simulink model "F28379DFirmware"  (R2026a)
settings: Solver=FixedStepAuto  StopTime=Inf  FixedStep=5e-5  EnableMultiTasking=on
undefined symbols (not defined in the file): bit, DiscIntNeverNeededParam, Down, F28379D_ADC_MaxCount, F28379D_ADC_Vmax, F28379D_PWM_Counter_Period, Foc_Ki_IxTcpu, Foc_Ki_S, Foc_Kp_I, Foc_Kp_S, GPTRIP1SEL, GPTRIP2SEL, Ia_offset, Ib_offset, IO334_DAC_Vmax, Maxon_645604_Np, PU_System_I_base, PU_System_N_base, Ts_CPU, TZ1, TZ2, Up
libraries: c280xlib x8, mcbcontrolslib x8, canmsglib x7, c2802xlib x6, mcbeeMathTransformLib x3, slpidlib x3, simulink x3, mcbpositiondecoderlib x3, c2837xDlib x3, demo_controls x1
(part 2 of 2)

== system F28379DFirmware/F28379D Firmware/Controller Algorithm/FOC/Speed Control MLD ==
  En_closedloop : Inport
  EnablePWM : Inport  Port=2
  SpeedRef : Inport  Port=3
  Speed_Meas_PU : Inport  Port=4
  Kp_S : Inport  Port=5
  Ki_S : Inport  Port=6
  AND : Logic  IconShape=distinctive  AllPortsSameDT=off  OutDataTypeStr=boolean
  Id_Ref : Constant  Value=0  OutDataTypeStr=single
  Mux : Mux  Inputs=2
  PI_Controller_Speed : Subsystem
  Speed_Ref_Selector : Subsystem
  IdqRef_PU : Outport  VectorParamsAs1DForOutWhenUnconnected=off
  wires:
  Mux/1 -> IdqRef_PU/1
  En_closedloop/1 -> AND/1, PI_Controller_Speed/1(Enable)
  Kp_S/1 -> PI_Controller_Speed/4(Kp_S)
  EnablePWM/1 -> AND/2
  Speed_Ref_Selector/1(Speed_Ref_PU) -> PI_Controller_Speed/2(N_ref)
  PI_Controller_Speed/1(Iq_ref) -> Mux/2
  SpeedRef/1 -> Speed_Ref_Selector/2(SpeedCommand)
  AND/1 -> Speed_Ref_Selector/1(Enable)
  Speed_Meas_PU/1 -> PI_Controller_Speed/3(N_fb), Speed_Ref_Selector/3(Speed_Ref_Open)
  Id_Ref/1 -> Mux/1
  Ki_S/1 -> PI_Controller_Speed/5(Ki_S)

== system F28379DFirmware/F28379D Firmware/Controller Algorithm/Speed and Pos Decoder/IndexFinder ==
  In1 : Inport
  Enable : EnablePort
  AND : Logic  AllPortsSameDT=off  OutDataTypeStr=boolean
  Compare To Constant : simulink/Logic and Bit Operations/Compare To Constant  relop===  const=0  OutDataTypeStr=boolean
  Compare To Constant1 : simulink/Logic and Bit Operations/Compare To Constant  relop=>  const=0  OutDataTypeStr=boolean
  Delay3 : Delay  DelayLength=1
  IndexFound : Outport
  wires:
  In1/1 -> Delay3/1, Compare To Constant1/1
  Compare To Constant1/1 -> AND/2
  Compare To Constant/1 -> AND/1
  Delay3/1 -> Compare To Constant/1
  AND/1 -> IndexFound/1

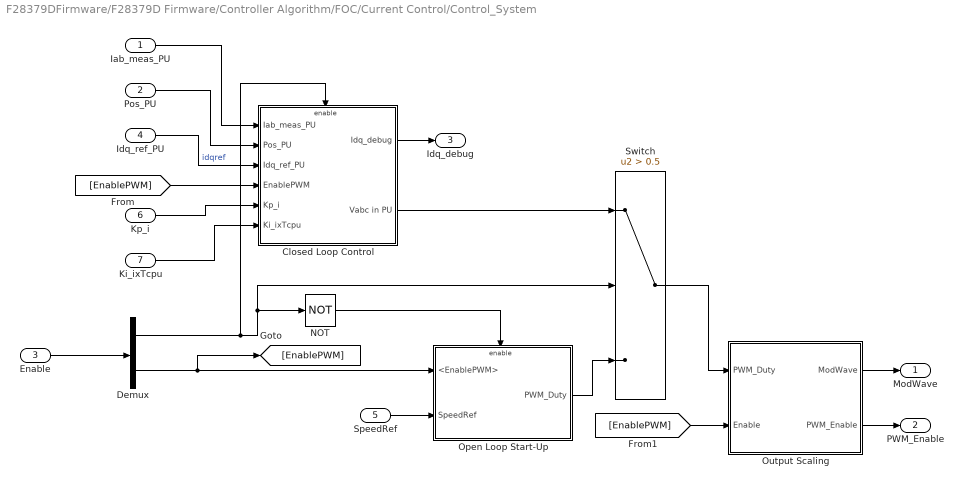
== system F28379DFirmware/F28379D Firmware/Controller Algorithm/FOC/Current Control/Control_System ==
  Iab_meas_PU : Inport
  Pos_PU : Inport  Port=2
  Enable : Inport  Port=3
  Idq_ref_PU : Inport  Port=4
  SpeedRef : Inport  Port=5
  Kp_i : Inport  Port=6
  Ki_ixTcpu : Inport  Port=7
  Closed Loop Control : Subsystem
  Demux : Demux  Outputs=2
  NOT : Logic  Operator=NOT  IconShape=distinctive  AllPortsSameDT=off  OutDataTypeStr=boolean
  Open Loop Start-Up : Subsystem
  Output Scaling : Subsystem
  Switch : Switch  Criteria=u2 > Threshold  Threshold=0.5  SaturateOnIntegerOverflow=off  InputSameDT=off
  ModWave : Outport
  PWM_Enable : Outport  Port=2
  Idq_debug : Outport  Port=3  VectorParamsAs1DForOutWhenUnconnected=off
  wires:
  Enable/1 -> Demux/1
  Idq_ref_PU/1 -> Closed Loop Control/3(Idq_ref_PU)  "idqref"
  Demux/2 -> [EnablePWM], Open Loop Start-Up/1(<EnablePWM>)
  [EnablePWM] -> Closed Loop Control/4(EnablePWM)
  Demux/1 -> Switch/2, NOT/1, Closed Loop Control/Enable
  Iab_meas_PU/1 -> Closed Loop Control/1(Iab_meas_PU)
  Pos_PU/1 -> Closed Loop Control/2(Pos_PU)
  SpeedRef/1 -> Open Loop Start-Up/2(SpeedRef)
  Kp_i/1 -> Closed Loop Control/5(Kp_i)
  Ki_ixTcpu/1 -> Closed Loop Control/6(Ki_ixTcpu)
  Closed Loop Control/2(Vabc in PU) -> Switch/1
  Closed Loop Control/1(Idq_debug) -> Idq_debug/1
  NOT/1 -> Open Loop Start-Up/Enable
  Open Loop Start-Up/1(PWM_Duty) -> Switch/3
  Switch/1 -> Output Scaling/1(PWM_Duty)
  [EnablePWM] -> Output Scaling/2(Enable)
  Output Scaling/2(PWM_Enable) -> PWM_Enable/1
  Output Scaling/1(ModWave) -> ModWave/1

== system F28379DFirmware/F28379D Firmware/Controller Algorithm/FOC/Speed Control MLD/PI_Controller_Speed ==
  Enable : Inport
  N_ref : Inport  Port=2
  N_fb : Inport  Port=3
  Kp_S : Inport  Port=4
  Ki_S : Inport  Port=5
  Discrete PI Controller with anti-windup & reset : slpidlib/PID Controller  Controller=PI  Form=Parallel  TimeDomain=Discrete-time  UseExternalTs=off  SampleTime=-1  IntegratorMethod=Forward Euler  FilterMethod=Forward Euler  ControllerParametersSource=external  P=1  I=1  UseKiTs=on  D=0  UseExternalDerivativeSource=off  N=100  UseFilter=on  TunerSelectOption=Transfer Function Based (PID Tuner App)  InitialConditionSource=external  InitialConditionForIntegrator=0  InitialConditionForFilter=0  DifferentiatorICPrevScaledInput=0  ExternalReset=level  TrackingMode=off  Kt=1  LimitOutput=on  SatLimitsSource=internal  UpperSaturationLimit=1  LowerSaturationLimit=-1  LinearizeAsGain=on  AntiWindupMode=clamping  Kb=1  LimitIntegrator=off  UpperIntegratorSaturationLimit=inf  LowerIntegratorSaturationLimit=-inf  RndMeth=Simplest  POutMin=[]  POutMax=[]  IOutMin=[]  IOutMax=[]  DOutMin=[]  DOutMax=[]  NOutMin=[]  NOutMax=[]  SumOutMin=[]  SumOutMax=[]  SaturationOutDataTypeStr=Inherit: Inherit via back propagation  SaturationOutMin=[]  SaturationOutMax=[]  PParamMin=[]  PParamMax=[]  IParamMin=[]  IParamMax=[]  DParamMin=[]  DParamMax=[]  NParamMin=[]  NParamMax=[]  KbParamMin=[]  KbParamMax=[]  KtParamMin=[]  KtParamMax=[]  KbOutMin=[]  KbOutMax=[]  KtOutMin=[]  KtOutMax=[]  IntegratorOutMin=[]  IntegratorOutMax=[]  FilterOutMin=[]  FilterOutMax=[]  SumI1OutMin=[]  SumI1OutMax=[]  SumI2OutMin=[]  SumI2OutMax=[]  SumI3OutMin=[]  SumI3OutMax=[]  SumI4OutMin=[]  SumI4OutMax=[]  SumDOutMin=[]  SumDOutMax=[]  DifferentiatorOutMin=[]  DifferentiatorOutMax=[]  FilterDiffOutCoefMin=[]  FilterDiffOutCoefMax=[]  ReciprocalOutMin=[]  ReciprocalOutMax=[]  SumDenOutMin=[]  SumDenOutMax=[]  SumNumOutMin=[]  SumNumOutMax=[]  DivideOutMin=[]  DivideOutMax=[]  UdiffTsProdOutMin=[]  UdiffTsProdOutMax=[]  NTsProdOutMin=[]  NTsProdOutMax=[]  UintegralTsProdOutMin=[]  UintegralTsProdOutMax=[]  UngainTsProdOutMin=[]  UngainTsProdOutMax=[]  ClampingZeroOutDataTypeStr=Inherit: Inherit via back propagation  ClampingZeroOutMin=[]  ClampingZeroOutMax=[]  FilterDenConstantOutDataTypeStr=Inherit: Inherit via back propagation  FilterDenConstantOutMin=[]  FilterDenConstantOutMax=[]  PCopyOutDataTypeStr=Inherit: Inherit via back propagation  PCopyOutMin=[]  PCopyOutMax=[]  NCopyOutDataTypeStr=Inherit: Inherit via back propagation  NCopyOutMin=[]  NCopyOutMax=[]  IntegratorContinuousStateAttributes=''  IntegratorStateMustResolveToSignalObject=off  IntegratorRTWStateStorageClass=Auto  FilterContinuousStateAttributes=''  FilterStateMustResolveToSignalObject=off  FilterRTWStateStorageClass=Auto  ParallelPVariant=ExternalParameters  IdealPVariant=Disabled  IVariant=ExternalParameters  DVariant=Disabled  IntegratorVariant=Discrete  SatVariant=Enabled  AWVariant=DiscClampingParallel  PCopyVariant=Disabled  TRVariant=Disabled  FdbkBlocksVariant=Forward  IdealPFdbkVariant=Disabled  SatFdbkVariant=Disabled  DerivativeFilterVariant=Disabled  NVariant=Disabled  NCopyVariant=Disabled_SignalSpec  FilterICVariant=Disabled  IntegratorICVariant=ExternalICs  ExternalResetVariant=ExternalReset  TRSumVariant=Passthrough  SumFdbkVariant=Disabled  SumVariant=Sum_PI  TsampFilterVariant=InternalTs  TsampNgainVariant=Passthrough  TsampIntegralVariant=Disabled_SignalSpec  ExternalSaturationOutDataTypeStr=Inherit: Same as second input  DerivativeSourceVariant=Disabled  PreIntVariant=InternalPreInt
  Ki2 : Constant  Value=0  OutDataTypeStr=single  SampleTime=-1
  Logical Operator : Logic  Operator=NOT  IconShape=distinctive  AllPortsSameDT=off  OutDataTypeStr=boolean
  Sum : Sum  Inputs=|+-  OutDataTypeStr=Inherit: Same as first input
  Iq_ref : Outport  VectorParamsAs1DForOutWhenUnconnected=off
  wires:
  Ki_S/1 -> Discrete PI Controller with anti-windup & reset/3
  Kp_S/1 -> Discrete PI Controller with anti-windup & reset/2
  Enable/1 -> Logical Operator/1
  Ki2/1 -> Discrete PI Controller with anti-windup & reset/5
  Logical Operator/1 -> Discrete PI Controller with anti-windup & reset/4
  Sum/1 -> Discrete PI Controller with anti-windup & reset/1
  N_ref/1 -> Sum/1
  N_fb/1 -> Sum/2
  Discrete PI Controller with anti-windup & reset/1 -> Iq_ref/1

== system F28379DFirmware/F28379D Firmware/Controller Algorithm/FOC/Speed Control MLD/Speed_Ref_Selector ==
  Enable : Inport
  SpeedCommand : Inport  Port=2
  Speed_Ref_Open : Inport  Port=3
  IIR Filter : mcbcontrolslib/IIR Filter  VariantControl=Low Pass Filter  VariantSelect=Low-pass  FilterConstantInputType=Specify via dialog  Filter_constant=0.01  InitialOutput=Specify via dialog  InitialOutputValue=0  ExternalReset=none  advancedSettings=off  Ts=50e-6  cutOff_freq=32.1525
  Switch : Switch  Criteria=u2 > Threshold  Threshold=0.5  SaturateOnIntegerOverflow=off  InputSameDT=off
  Speed_Ref_PU : Outport
  wires:
  SpeedCommand/1 -> Switch/1  "SpeedRef"
  Enable/1 -> Switch/2
  Speed_Ref_Open/1 -> Switch/3
  Switch/1 -> IIR Filter/1
  IIR Filter/1 -> Speed_Ref_PU/1

== system F28379DFirmware/F28379D Firmware/Controller Algorithm/FOC/Current Control/Control_System/Closed Loop Control ==
  Iab_meas_PU : Inport
  Pos_PU : Inport  Port=2
  Idq_ref_PU : Inport  Port=3
  EnablePWM : Inport  Port=4
  Kp_i : Inport  Port=5
  Ki_ixTcpu : Inport  Port=6
  Enable : EnablePort
  Subsystem : Subsystem
  Terminator : Terminator
  Idq_debug : Outport
  Vabc in PU : Outport  Port=2
  wires:
  Subsystem/3(VI_fb) -> Terminator/1
  Idq_ref_PU/1 -> Subsystem/3(Idq_ref_PU)
  Iab_meas_PU/1 -> Subsystem/1(Iab_meas_PU)
  EnablePWM/1 -> Subsystem/4(EnablePWM)
  Pos_PU/1 -> Subsystem/2(Pos_PU)
  Subsystem/2(VIdq_debug) -> Idq_debug/1
  Subsystem/1(Vabc in PU) -> Vabc in PU/1
  Ki_ixTcpu/1 -> Subsystem/6(Ki_ixTcpu)
  Kp_i/1 -> Subsystem/5(Kp_i)

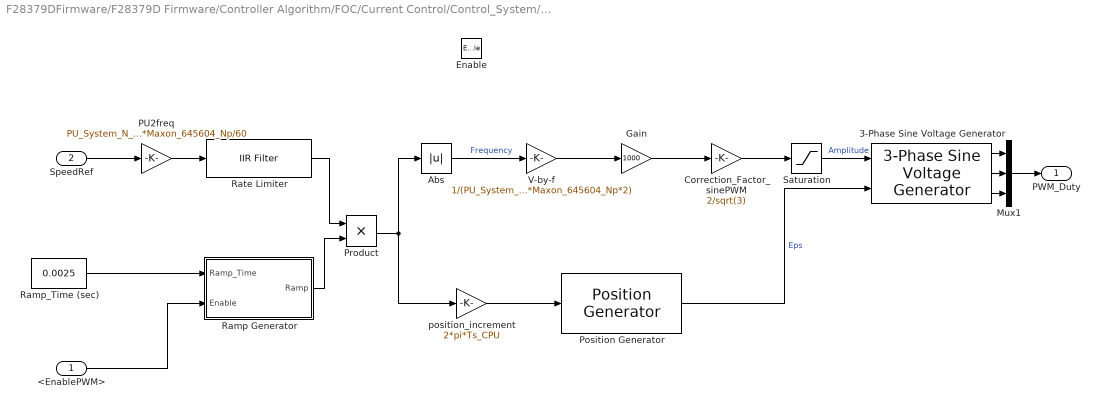
== system F28379DFirmware/F28379D Firmware/Controller Algorithm/FOC/Current Control/Control_System/Open Loop Start-Up ==
  <EnablePWM> : Inport
  SpeedRef : Inport  Port=2
  Enable : EnablePort
  3-Phase Sine Voltage Generator : mcbcontrolslib/3-Phase Sine Voltage Generator  AngleInput=Radians  N_points=1024
  Abs : Abs  SaturateOnIntegerOverflow=off
  Correction_Factor_sinePWM : Gain  Gain=2/sqrt(3)  RndMeth=Simplest  OutDataTypeStr=Inherit: Same as input
  Gain : Gain  Gain=1000
  Mux1 : Mux  Inputs=3
  PU2freq : Gain  Gain=PU_System_N_base *Maxon_645604_Np/60  RndMeth=Simplest  OutDataTypeStr=Inherit: Same as input
  Position Generator : mcbcontrolslib/Position Generator  AngleOutput=Radians  InitialThetaSource=Specify via dialog  ExternalReset=none  Offset=0
  Product : Product  RndMeth=Simplest  OutDataTypeStr=Inherit: Same as first input
  Ramp Generator : Subsystem
  Ramp_Time (sec) : Constant  Value=0.0025  OutDataTypeStr=single  SampleTime=-1
  Rate Limiter : mcbcontrolslib/IIR Filter  VariantControl=Low Pass Filter  VariantSelect=Low-pass  FilterConstantInputType=Specify via dialog  Filter_constant=0.0001  InitialOutput=Specify via dialog  InitialOutputValue=0  ExternalReset=none  advancedSettings=off  Ts=50e-6  cutOff_freq=0.31834
  Saturation : Saturate  UpperLimit=0.95  LowerLimit=0.15  RndMeth=Simplest
  V-by-f : Gain  Gain=1/(PU_System_N_base*Maxon_645604_Np*2)  RndMeth=Simplest  OutDataTypeStr=Inherit: Same as input
  position_increment : Gain  Gain=2*pi*Ts_CPU  RndMeth=Simplest  OutDataTypeStr=Inherit: Same as input
  PWM_Duty : Outport  VectorParamsAs1DForOutWhenUnconnected=off
  wires:
  3-Phase Sine Voltage Generator/1 -> Mux1/1
  3-Phase Sine Voltage Generator/3 -> Mux1/3
  Position Generator/1 -> 3-Phase Sine Voltage Generator/2  "Eps"
  Saturation/1 -> 3-Phase Sine Voltage Generator/1  "Amplitude"
  Mux1/1 -> PWM_Duty/1
  Ramp Generator/1(Ramp) -> Product/2
  Ramp_Time (sec)/1 -> Ramp Generator/1(Ramp_Time)
  Abs/1 -> V-by-f/1  "Frequency"
  position_increment/1 -> Position Generator/1
  V-by-f/1 -> Gain/1
  PU2freq/1 -> Rate Limiter/1
  Correction_Factor_sinePWM/1 -> Saturation/1
  3-Phase Sine Voltage Generator/2 -> Mux1/2
  <EnablePWM>/1 -> Ramp Generator/2(Enable)
  Product/1 -> Abs/1, position_increment/1
  Rate Limiter/1 -> Product/1
  SpeedRef/1 -> PU2freq/1
  Gain/1 -> Correction_Factor_sinePWM/1

== system F28379DFirmware/F28379D Firmware/Controller Algorithm/FOC/Current Control/Control_System/Output Scaling ==
  PWM_Duty : Inport
  Enable : Inport  Port=2
  Constant : Constant  Value=0.5  OutDataTypeStr=single
  Data Type Conversion : DataTypeConversion  OutDataTypeStr=single  SaturateOnIntegerOverflow=off  RndMeth=Floor
  Gain : Gain  Gain=0.5  OutDataTypeStr=Inherit: Same as input
  Sum : Sum  Inputs=|++
  ModWave : Outport
  PWM_Enable : Outport  Port=2
  wires:
  Sum/1 -> ModWave/1  "duty"
  Constant/1 -> Sum/2
  Gain/1 -> Sum/1  "ModWave"
  PWM_Duty/1 -> Gain/1
  Data Type Conversion/1 -> PWM_Enable/1
  Enable/1 -> Data Type Conversion/1

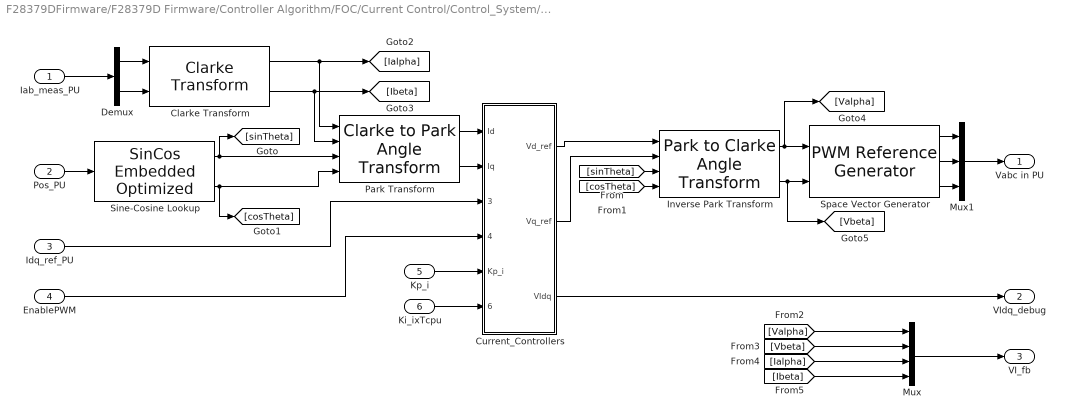
== system F28379DFirmware/F28379D Firmware/Controller Algorithm/FOC/Current Control/Control_System/Closed Loop Control/Subsystem ==
  Iab_meas_PU : Inport
  Pos_PU : Inport  Port=2
  Idq_ref_PU : Inport  Port=3
  EnablePWM : Inport  Port=4
  Kp_i : Inport  Port=5
  Ki_ixTcpu : Inport  Port=6
  Clarke Transform : mcbeeMathTransformLib/Clarke Transform  VariantControl=Variant2  PowerInvariant=off  UseWithEmbedded=on  PhaseInput=Two inputs
      settings: LibrarySourceBlock=mcbcontrolslib/Clarke Transform
  Current_Controllers : Subsystem
  Demux : Demux  Outputs=2
  Inverse Park Transform : mcbeeMathTransformLib/Park to Clarke Angle Transform  AxisAlignment=D-axis  UseWithEmbedded=on  PhaseInput=Two inputs  ThetaInput=Sine and Cosine electrical position  AngleInput=Per-unit  N_points=1024
      settings: LibrarySourceBlock=mcbcontrolslib/Inverse Park Transform
  Mux : Mux
  Mux1 : Mux  Inputs=3
  Park Transform : mcbeeMathTransformLib/Clarke to Park Angle Transform  AxisAlignment=D-axis  UseWithEmbedded=on  PhaseInput=Two inputs  ThetaInput=Sine and Cosine electrical position  AngleInput=Per-unit  N_points=1024
      settings: LibrarySourceBlock=mcbcontrolslib/Park Transform
  Sine-Cosine Lookup : mcbcontrolslib/SinCos Embedded Optimized  LabelModeActiveChoice=MCB_Sin  OptforProc=off  OptLevelPop=Disabled  ApproximationMethod=None  UserApproxMethod=Lookup  ApproxStatus=None  ThetaDataType=double  CopyThetaDataType=single  InterpMethod=Linear point-slope  NumberOfDataPoints=16  NumberOfIterations=11  RemoveProtectionAgainstOutOfRangeInput=off  TableDataTypeStr=Inherit: Inherit via input  AngleInput=Per-unit  CopyAngleInput=Per-unit  N_points=1024  CopyN_points=1024  Datatype=single  CopyTableDatatype=Inherit: Same as input  DatatypeInput=Inherit from input  IsPrevStrictOpt=0  IsPrevLUTForced=0
  Space Vector Generator : mcbcontrolslib/PWM Reference Generator  modType=SVM: space vector modulation  inSignal=Valphabeta  expandVoltageInput=on  inputUnits=Per-unit  LimitModulation=off  enableVoltage=on  enableModulationSignal=off  enableDutyCycle=off  expandVoltageOutput=on
  Vabc in PU : Outport  VectorParamsAs1DForOutWhenUnconnected=off
  VIdq_debug : Outport  Port=2  VectorParamsAs1DForOutWhenUnconnected=off
  VI_fb : Outport  Port=3
  wires:
  Space Vector Generator/2 -> Mux1/2
  Clarke Transform/2 -> [Ibeta], Park Transform/2
  Idq_ref_PU/1 -> Current_Controllers/3(Idq_ref_PU)
  Park Transform/1 -> Current_Controllers/1(Id)
  Current_Controllers/1(Vd_ref) -> Inverse Park Transform/1
  Clarke Transform/1 -> [Ialpha], Park Transform/1
  Space Vector Generator/1 -> Mux1/1
  Iab_meas_PU/1 -> Demux/1
  Inverse Park Transform/1 -> [Valpha], Space Vector Generator/1
  Sine-Cosine Lookup/2 -> Park Transform/4, [cosTheta]
  Demux/2 -> Clarke Transform/2
  [sinTheta] -> Inverse Park Transform/3
  Park Transform/2 -> Current_Controllers/2(Iq)
  Current_Controllers/3(VIdq) -> VIdq_debug/1
  Mux1/1 -> Vabc in PU/1
  Sine-Cosine Lookup/1 -> Park Transform/3, [sinTheta]
  Demux/1 -> Clarke Transform/1
  Current_Controllers/2(Vq_ref) -> Inverse Park Transform/2
  [cosTheta] -> Inverse Park Transform/4
  Space Vector Generator/3 -> Mux1/3
  EnablePWM/1 -> Current_Controllers/4(EnablePWM)
  [Valpha] -> Mux/1
  Mux/1 -> VI_fb/1
  Pos_PU/1 -> Sine-Cosine Lookup/1
  Inverse Park Transform/2 -> [Vbeta], Space Vector Generator/2
  [Ialpha] -> Mux/3
  [Ibeta] -> Mux/4
  [Vbeta] -> Mux/2
  Ki_ixTcpu/1 -> Current_Controllers/6(Ki_ixTcpu)
  Kp_i/1 -> Current_Controllers/5(Kp_i)

== system F28379DFirmware/F28379D Firmware/Controller Algorithm/FOC/Current Control/Control_System/Open Loop Start-Up/Ramp Generator ==
  Ramp_Time : Inport
  Enable : Inport  Port=2
  Divide : Product  Inputs=*/  RndMeth=Simplest  OutDataTypeStr=Inherit: Same as first input
  NOT : Logic  Operator=NOT  IconShape=distinctive  AllPortsSameDT=off  OutDataTypeStr=boolean
  One : Constant  OutDataTypeStr=single  SampleTime=-1
  Ramp Generator : DiscreteIntegrator  IntegratorMethod=Accumulation: Forward Euler  gainval=1  ExternalReset=sampled level  SampleTime=-1  OutDataTypeStr=single  RndMeth=Simplest  LimitOutput=on  UpperSaturationLimit=1  LowerSaturationLimit=0  ICPrevOutput=DiscIntNeverNeededParam  ICPrevScaledInput=DiscIntNeverNeededParam
  Sample_Time : Gain  Gain=Ts_CPU  RndMeth=Simplest  OutDataTypeStr=Inherit: Same as input
  Ramp : Outport
  wires:
  Divide/1 -> Sample_Time/1
  Ramp Generator/1 -> Ramp/1  "Eps"
  Sample_Time/1 -> Ramp Generator/1
  One/1 -> Divide/1
  Ramp_Time/1 -> Divide/2
  Enable/1 -> NOT/1
  NOT/1 -> Ramp Generator/2

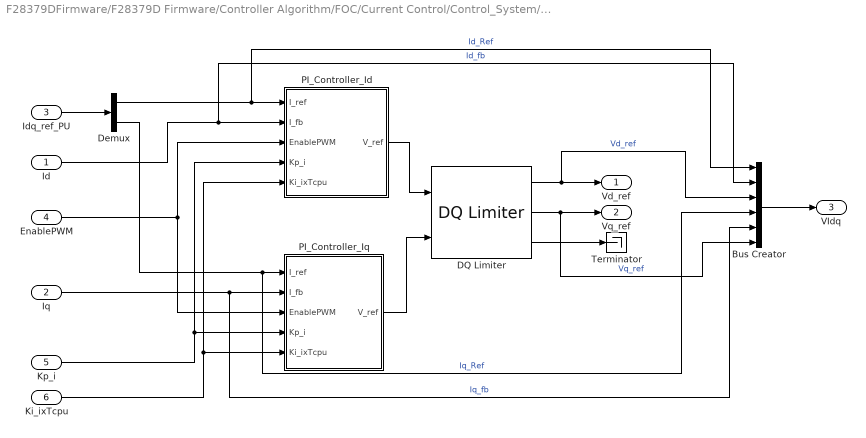
== system F28379DFirmware/F28379D Firmware/Controller Algorithm/FOC/Current Control/Control_System/Closed Loop Control/Subsystem/Current_Controllers ==
  Id : Inport
  Iq : Inport  Port=2
  Idq_ref_PU : Inport  Port=3
  EnablePWM : Inport  Port=4
  Kp_i : Inport  Port=5
  Ki_ixTcpu : Inport  Port=6
  Bus Creator : BusCreator  Inputs=6
  DQ Limiter : mcbcontrolslib/DQ Limiter  satMethodInputType=Specify via dialog  satMethodSelected=D-Q equivalence  satLimitInputType=Specify via dialog  Vmax=0.95
  Demux : Demux  Outputs=2
  PI_Controller_Id : Subsystem
  PI_Controller_Iq : Subsystem
  Terminator : Terminator
  Vd_ref : Outport  VectorParamsAs1DForOutWhenUnconnected=off
  Vq_ref : Outport  Port=2  VectorParamsAs1DForOutWhenUnconnected=off
  VIdq : Outport  Port=3  VectorParamsAs1DForOutWhenUnconnected=off
  wires:
  Iq/1 -> Bus Creator/5, PI_Controller_Iq/2(I_fb)  "Iq_fb"
  Id/1 -> Bus Creator/2, PI_Controller_Id/2(I_fb)  "Id_fb"
  Demux/1 -> Bus Creator/1, PI_Controller_Id/1(I_ref)  "Id_Ref"
  Demux/2 -> Bus Creator/4, PI_Controller_Iq/1(I_ref)  "Iq_Ref"
  Idq_ref_PU/1 -> Demux/1
  PI_Controller_Id/1(V_ref) -> DQ Limiter/1
  PI_Controller_Iq/1(V_ref) -> DQ Limiter/2
  DQ Limiter/1 -> Vd_ref/1, Bus Creator/3  "Vd_ref"
  DQ Limiter/2 -> Vq_ref/1, Bus Creator/6  "Vq_ref"
  DQ Limiter/3 -> Terminator/1
  Bus Creator/1 -> VIdq/1
  EnablePWM/1 -> PI_Controller_Iq/3(EnablePWM), PI_Controller_Id/3(EnablePWM)
  Kp_i/1 -> PI_Controller_Iq/4(Kp_i), PI_Controller_Id/4(Kp_i)
  Ki_ixTcpu/1 -> PI_Controller_Iq/5(Ki_ixTcpu), PI_Controller_Id/5(Ki_ixTcpu)

== system F28379DFirmware/F28379D Firmware/Controller Algorithm/FOC/Current Control/Control_System/Closed Loop Control/Subsystem/Current_Controllers/PI_Controller_Id ==
  I_ref : Inport
  I_fb : Inport  Port=2
  EnablePWM : Inport  Port=3
  Kp_i : Inport  Port=4
  Ki_ixTcpu : Inport  Port=5
  Discrete PI Controller with anti-windup & reset : slpidlib/PID Controller  Controller=PI  Form=Parallel  TimeDomain=Discrete-time  UseExternalTs=off  SampleTime=-1  IntegratorMethod=Forward Euler  FilterMethod=Forward Euler  ControllerParametersSource=external  P=1  I=1  UseKiTs=on  D=0  UseExternalDerivativeSource=off  N=100  UseFilter=on  TunerSelectOption=Transfer Function Based (PID Tuner App)  InitialConditionSource=external  InitialConditionForIntegrator=0  InitialConditionForFilter=0  DifferentiatorICPrevScaledInput=0  ExternalReset=level  TrackingMode=off  Kt=1  LimitOutput=on  SatLimitsSource=internal  UpperSaturationLimit=1  LowerSaturationLimit=-1  LinearizeAsGain=on  AntiWindupMode=clamping  Kb=1  LimitIntegrator=off  UpperIntegratorSaturationLimit=inf  LowerIntegratorSaturationLimit=-inf  RndMeth=Simplest  POutMin=[]  POutMax=[]  IOutMin=[]  IOutMax=[]  DOutMin=[]  DOutMax=[]  NOutMin=[]  NOutMax=[]  SumOutMin=[]  SumOutMax=[]  SaturationOutDataTypeStr=Inherit: Inherit via back propagation  SaturationOutMin=[]  SaturationOutMax=[]  PParamMin=[]  PParamMax=[]  IParamMin=[]  IParamMax=[]  DParamMin=[]  DParamMax=[]  NParamMin=[]  NParamMax=[]  KbParamMin=[]  KbParamMax=[]  KtParamMin=[]  KtParamMax=[]  KbOutMin=[]  KbOutMax=[]  KtOutMin=[]  KtOutMax=[]  IntegratorOutMin=[]  IntegratorOutMax=[]  FilterOutMin=[]  FilterOutMax=[]  SumI1OutMin=[]  SumI1OutMax=[]  SumI2OutMin=[]  SumI2OutMax=[]  SumI3OutMin=[]  SumI3OutMax=[]  SumI4OutMin=[]  SumI4OutMax=[]  SumDOutMin=[]  SumDOutMax=[]  DifferentiatorOutMin=[]  DifferentiatorOutMax=[]  FilterDiffOutCoefMin=[]  FilterDiffOutCoefMax=[]  ReciprocalOutMin=[]  ReciprocalOutMax=[]  SumDenOutMin=[]  SumDenOutMax=[]  SumNumOutMin=[]  SumNumOutMax=[]  DivideOutMin=[]  DivideOutMax=[]  UdiffTsProdOutMin=[]  UdiffTsProdOutMax=[]  NTsProdOutMin=[]  NTsProdOutMax=[]  UintegralTsProdOutMin=[]  UintegralTsProdOutMax=[]  UngainTsProdOutMin=[]  UngainTsProdOutMax=[]  ClampingZeroOutDataTypeStr=Inherit: Inherit via back propagation  ClampingZeroOutMin=[]  ClampingZeroOutMax=[]  FilterDenConstantOutDataTypeStr=Inherit: Inherit via back propagation  FilterDenConstantOutMin=[]  FilterDenConstantOutMax=[]  PCopyOutDataTypeStr=Inherit: Inherit via back propagation  PCopyOutMin=[]  PCopyOutMax=[]  NCopyOutDataTypeStr=Inherit: Inherit via back propagation  NCopyOutMin=[]  NCopyOutMax=[]  IntegratorContinuousStateAttributes=''  IntegratorStateMustResolveToSignalObject=off  IntegratorRTWStateStorageClass=Auto  FilterContinuousStateAttributes=''  FilterStateMustResolveToSignalObject=off  FilterRTWStateStorageClass=Auto  ParallelPVariant=ExternalParameters  IdealPVariant=Disabled  IVariant=ExternalParameters  DVariant=Disabled  IntegratorVariant=Discrete  SatVariant=Enabled  AWVariant=DiscClampingParallel  PCopyVariant=Disabled  TRVariant=Disabled  FdbkBlocksVariant=Forward  IdealPFdbkVariant=Disabled  SatFdbkVariant=Disabled  DerivativeFilterVariant=Disabled  NVariant=Disabled  NCopyVariant=Disabled_SignalSpec  FilterICVariant=Disabled  IntegratorICVariant=ExternalICs  ExternalResetVariant=ExternalReset  TRSumVariant=Passthrough  SumFdbkVariant=Disabled  SumVariant=Sum_PI  TsampFilterVariant=InternalTs  TsampNgainVariant=Passthrough  TsampIntegralVariant=Disabled_SignalSpec  ExternalSaturationOutDataTypeStr=Inherit: Same as second input  DerivativeSourceVariant=Disabled  PreIntVariant=InternalPreInt
  Ki1 : Constant  Value=0  OutDataTypeStr=single  SampleTime=-1
  Logical Operator : Logic  Operator=NOT  IconShape=distinctive  AllPortsSameDT=off  OutDataTypeStr=boolean
  Sum : Sum  Inputs=|+-  OutDataTypeStr=Inherit: Same as first input
  V_ref : Outport  VectorParamsAs1DForOutWhenUnconnected=off
  wires:
  I_ref/1 -> Sum/1
  I_fb/1 -> Sum/2
  Discrete PI Controller with anti-windup & reset/1 -> V_ref/1
  Sum/1 -> Discrete PI Controller with anti-windup & reset/1
  Logical Operator/1 -> Discrete PI Controller with anti-windup & reset/4
  Ki1/1 -> Discrete PI Controller with anti-windup & reset/5
  EnablePWM/1 -> Logical Operator/1
  Kp_i/1 -> Discrete PI Controller with anti-windup & reset/2
  Ki_ixTcpu/1 -> Discrete PI Controller with anti-windup & reset/3

== system F28379DFirmware/F28379D Firmware/Controller Algorithm/FOC/Current Control/Control_System/Closed Loop Control/Subsystem/Current_Controllers/PI_Controller_Iq ==
  I_ref : Inport
  I_fb : Inport  Port=2
  EnablePWM : Inport  Port=3
  Kp_i : Inport  Port=4
  Ki_ixTcpu : Inport  Port=5
  Discrete PI Controller with anti-windup & reset : slpidlib/PID Controller  Controller=PI  Form=Parallel  TimeDomain=Discrete-time  UseExternalTs=off  SampleTime=-1  IntegratorMethod=Forward Euler  FilterMethod=Forward Euler  ControllerParametersSource=external  P=1  I=1  UseKiTs=on  D=0  UseExternalDerivativeSource=off  N=100  UseFilter=on  TunerSelectOption=Transfer Function Based (PID Tuner App)  InitialConditionSource=external  InitialConditionForIntegrator=0  InitialConditionForFilter=0  DifferentiatorICPrevScaledInput=0  ExternalReset=level  TrackingMode=off  Kt=1  LimitOutput=on  SatLimitsSource=internal  UpperSaturationLimit=1  LowerSaturationLimit=-1  LinearizeAsGain=on  AntiWindupMode=clamping  Kb=1  LimitIntegrator=off  UpperIntegratorSaturationLimit=inf  LowerIntegratorSaturationLimit=-inf  RndMeth=Simplest  POutMin=[]  POutMax=[]  IOutMin=[]  IOutMax=[]  DOutMin=[]  DOutMax=[]  NOutMin=[]  NOutMax=[]  SumOutMin=[]  SumOutMax=[]  SaturationOutDataTypeStr=Inherit: Inherit via back propagation  SaturationOutMin=[]  SaturationOutMax=[]  PParamMin=[]  PParamMax=[]  IParamMin=[]  IParamMax=[]  DParamMin=[]  DParamMax=[]  NParamMin=[]  NParamMax=[]  KbParamMin=[]  KbParamMax=[]  KtParamMin=[]  KtParamMax=[]  KbOutMin=[]  KbOutMax=[]  KtOutMin=[]  KtOutMax=[]  IntegratorOutMin=[]  IntegratorOutMax=[]  FilterOutMin=[]  FilterOutMax=[]  SumI1OutMin=[]  SumI1OutMax=[]  SumI2OutMin=[]  SumI2OutMax=[]  SumI3OutMin=[]  SumI3OutMax=[]  SumI4OutMin=[]  SumI4OutMax=[]  SumDOutMin=[]  SumDOutMax=[]  DifferentiatorOutMin=[]  DifferentiatorOutMax=[]  FilterDiffOutCoefMin=[]  FilterDiffOutCoefMax=[]  ReciprocalOutMin=[]  ReciprocalOutMax=[]  SumDenOutMin=[]  SumDenOutMax=[]  SumNumOutMin=[]  SumNumOutMax=[]  DivideOutMin=[]  DivideOutMax=[]  UdiffTsProdOutMin=[]  UdiffTsProdOutMax=[]  NTsProdOutMin=[]  NTsProdOutMax=[]  UintegralTsProdOutMin=[]  UintegralTsProdOutMax=[]  UngainTsProdOutMin=[]  UngainTsProdOutMax=[]  ClampingZeroOutDataTypeStr=Inherit: Inherit via back propagation  ClampingZeroOutMin=[]  ClampingZeroOutMax=[]  FilterDenConstantOutDataTypeStr=Inherit: Inherit via back propagation  FilterDenConstantOutMin=[]  FilterDenConstantOutMax=[]  PCopyOutDataTypeStr=Inherit: Inherit via back propagation  PCopyOutMin=[]  PCopyOutMax=[]  NCopyOutDataTypeStr=Inherit: Inherit via back propagation  NCopyOutMin=[]  NCopyOutMax=[]  IntegratorContinuousStateAttributes=''  IntegratorStateMustResolveToSignalObject=off  IntegratorRTWStateStorageClass=Auto  FilterContinuousStateAttributes=''  FilterStateMustResolveToSignalObject=off  FilterRTWStateStorageClass=Auto  ParallelPVariant=ExternalParameters  IdealPVariant=Disabled  IVariant=ExternalParameters  DVariant=Disabled  IntegratorVariant=Discrete  SatVariant=Enabled  AWVariant=DiscClampingParallel  PCopyVariant=Disabled  TRVariant=Disabled  FdbkBlocksVariant=Forward  IdealPFdbkVariant=Disabled  SatFdbkVariant=Disabled  DerivativeFilterVariant=Disabled  NVariant=Disabled  NCopyVariant=Disabled_SignalSpec  FilterICVariant=Disabled  IntegratorICVariant=ExternalICs  ExternalResetVariant=ExternalReset  TRSumVariant=Passthrough  SumFdbkVariant=Disabled  SumVariant=Sum_PI  TsampFilterVariant=InternalTs  TsampNgainVariant=Passthrough  TsampIntegralVariant=Disabled_SignalSpec  ExternalSaturationOutDataTypeStr=Inherit: Same as second input  DerivativeSourceVariant=Disabled  PreIntVariant=InternalPreInt
  Kp1 : Constant  Value=0  OutDataTypeStr=single  SampleTime=-1
  Logical Operator : Logic  Operator=NOT  IconShape=distinctive  AllPortsSameDT=off  OutDataTypeStr=boolean
  Sum : Sum  Inputs=|+-  OutDataTypeStr=Inherit: Same as first input
  V_ref : Outport  VectorParamsAs1DForOutWhenUnconnected=off
  wires:
  Discrete PI Controller with anti-windup & reset/1 -> V_ref/1
  I_fb/1 -> Sum/2
  I_ref/1 -> Sum/1
  Sum/1 -> Discrete PI Controller with anti-windup & reset/1
  Logical Operator/1 -> Discrete PI Controller with anti-windup & reset/4
  Kp1/1 -> Discrete PI Controller with anti-windup & reset/5
  EnablePWM/1 -> Logical Operator/1
  Kp_i/1 -> Discrete PI Controller with anti-windup & reset/2
  Ki_ixTcpu/1 -> Discrete PI Controller with anti-windup & reset/3
